simulink model "LMS_WITH_DWT"  (R2016a)
settings: Solver=VariableStepAuto  StartTime=0.0  StopTime=4000  RelTol=1e-3
libraries: dspstat3 x2, dspmlti4 x1, dspsrcs4 x1, dspmathops x1
settings Model: Creator=HP  LastModifiedBy=HP

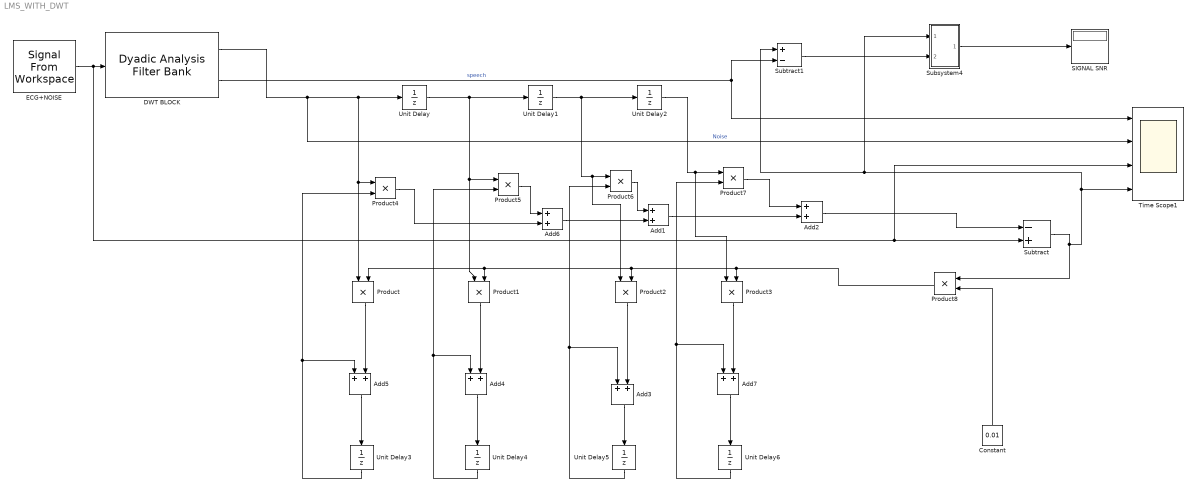
== system LMS_WITH_DWT ==
  Add{1..7} (7 alike) : Sum
  Constant : Constant  Value=0.01
  DWT BLOCK : dspmlti4/Dyadic Analysis Filter Bank  Wname=Discrete Meyer  OrdRec_ordDec=[1 / 1]  Order=2  LPF="[0.0352   -0.0854   -0.1350   0.4599   0.8069   0.3327]"  HPF="[-0.3327    0.8069   -0.4599   -0.1350    0.0854    0.0352]"  NumLevels=1  tree=Symmetric  Output=Multiple ports  OutputFrames=off
  ECG+NOISE : dspsrcs4/Signal From Workspace  X=y  Ts=1  nsamps=2  OutputAfterFinalValue=Setting to zero  ignoreOrWarnInputAndFrameLengths=off  OutputFrames=off
  Product{,1..8} (9 alike) : Product
  "SIGNAL SNR " : Display
  Subsystem4 : Subsystem
  Subtract : Sum  Inputs=-+
  Subtract1 : Sum  Inputs=+-
  Time Scope1 : Scope  NumInputPorts=4
  Unit Delay{,1..6} (7 alike) : UnitDelay  SampleTime=-1
  wires:
  Unit Delay/1 -> Product5/1, Product1/1, Unit Delay1/1
  Unit Delay1/1 -> Product2/1, Product6/1, Unit Delay2/1
  Unit Delay2/1 -> Product7/1, Product3/1
  DWT BLOCK/2 -> Subtract1/2, Time Scope1/1  "speech"
  Unit Delay3/1 -> Add5/1, Product4/2
  Product/1 -> Add5/2
  Product8/1 -> Product/2, Product1/2, Product2/2, Product3/2
  Unit Delay4/1 -> Add4/1, Product5/2
  Add5/1 -> Unit Delay3/1
  Add4/1 -> Unit Delay4/1
  Product1/1 -> Add4/2
  Product5/1 -> Add6/1
  Product4/1 -> Add6/2
  Product2/1 -> Add3/2
  Unit Delay5/1 -> Add3/1, Product6/2
  Add3/1 -> Unit Delay5/1
  Product6/1 -> Add1/1
  Add6/1 -> Add1/2
  Unit Delay6/1 -> Add7/1, Product7/2
  Product3/1 -> Add7/2
  Product7/1 -> Add2/1
  Add1/1 -> Add2/2
  Add7/1 -> Unit Delay6/1
  Constant/1 -> Product8/2
  ECG+NOISE/1 -> Time Scope1/3, Subtract/2, DWT BLOCK/1
  Add2/1 -> Subtract/1
  Subtract1/1 -> Subsystem4/2(In2)
  DWT BLOCK/1 -> Time Scope1/2, Product4/1, Product/1, Unit Delay/1  "Noise"
  Subtract/1 -> Product8/1, Time Scope1/4, Subsystem4/1(In1), Subtract1/1
  Subsystem4/1(Out1) -> "SIGNAL SNR "/1

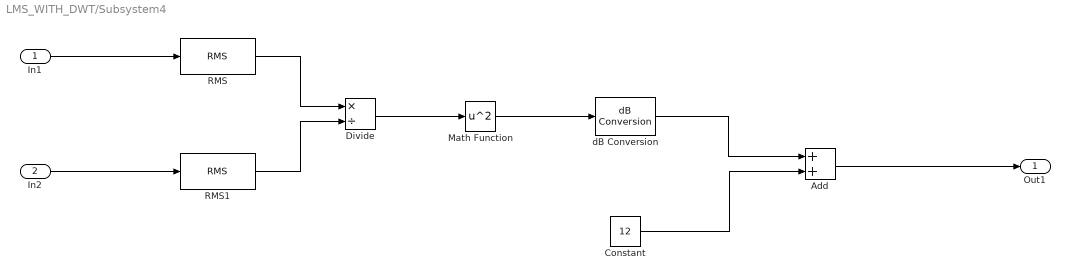
== system LMS_WITH_DWT/Subsystem4 ==
  In1 : Inport
  In2 : Inport  Port=2
  Add : Sum
  Constant : Constant  Value=12
  Divide : Product  Inputs=*/
  Math Function : Math  Operator=square  OutputSignalType=real  SaturateOnIntegerOverflow=on
  RMS : dspstat3/RMS  run=on  reset_popup=None  InputProcessing=Columns as channels (frame based)  directionMode=Each column  dimension=1
  RMS1 : dspstat3/RMS  run=on  reset_popup=None  InputProcessing=Columns as channels (frame based)  directionMode=Each column  dimension=1
  dB Conversion : dspmathops/dB Conversion  dBtype=dB  intype=Amplitude  R=1  fuzz=off
  Out1 : Outport
  wires:
  RMS1/1 -> Divide/2
  dB Conversion/1 -> Add/1
  In1/1 -> RMS/1
  Divide/1 -> Math Function/1
  RMS/1 -> Divide/1
  In2/1 -> RMS1/1
  Add/1 -> Out1/1
  Constant/1 -> Add/2
  Math Function/1 -> dB Conversion/1
